simulink model "HARMALYZE_model_simulink"  (R2019b)
settings: Solver=VariableStepAuto  StartTime=0.0  StopTime=2.3  RelTol=1e-3
libraries: powerlib_meascontrol x1
(part 2 of 2)

== system HARMALYZE_model_simulink/Subsystem2/Subsystem1/An Bn finder ==
  signal : Inport
  pulse : Inport  Port=2
  cos : Inport  Port=3
  sin : Inport  Port=4
  "freq " : Inport  Port=5
  Add2 : Sum  Inputs=+-
  Constant1 : Constant  Value=0.0095
  Data Store Read1 : DataStoreRead  DataStoreName=simultion_time
  Product : Product  Inputs=3
  Product{1,3..5} (4 alike) : Product
  Product2 : Product  Inputs=3
  Pulse Generator1 : DiscretePulseGenerator  PulseType=Time based  Period=1  PulseWidth=0.01
  Transfer Fcn1 : TransferFcn  Numerator=[2]  Denominator=[1 0]
  Transfer Fcn2 : TransferFcn  Numerator=[2]  Denominator=[1 0]
  Variable Time Delay1 : VariableTransportDelay  MaximumDelay=10
  An : Outport
  Bn : Outport  Port=2
  wires:
  Product4/1 -> Bn/1
  Product5/1 -> An/1
  Product3/1 -> Product4/2  "Bn"
  Add2/1 -> Variable Time Delay1/2
  Variable Time Delay1/1 -> Product4/1, Product5/2
  Data Store Read1/1 -> Add2/1
  Constant1/1 -> Add2/2
  Product1/1 -> Product5/1  "An"
  Pulse Generator1/1 -> Variable Time Delay1/1
  "freq "/1 -> Product3/1, Product1/2
  Transfer Fcn1/1 -> Product1/1
  Transfer Fcn2/1 -> Product3/2
  sin/1 -> Product2/3
  cos/1 -> Product/3
  Product2/1 -> Transfer Fcn2/1
  Product/1 -> Transfer Fcn1/1
  signal/1 -> Product/2, Product2/1
  pulse/1 -> Product2/2, Product/1

== system HARMALYZE_model_simulink/Subsystem2/Subsystem1/magnitude ==
  An : Inport
  Bn : Inport  Port=2
  Add3 : Sum
  Math Function : Math  Operator=square  SignedPower=off  SaturateOnIntegerOverflow=on
  Math Function1 : Math  Operator=square  SignedPower=off  SaturateOnIntegerOverflow=on
  Sqrt : Sqrt  SaturateOnIntegerOverflow=on
  Out1 : Outport
  wires:
  An/1 -> Math Function/1
  Bn/1 -> Math Function1/1
  Sqrt/1 -> Out1/1
  Math Function1/1 -> Add3/2
  Add3/1 -> Sqrt/1
  Math Function/1 -> Add3/1

== system HARMALYZE_model_simulink/Subsystem2/Subsystem1/phase ==
  An : Inport
  Bn : Inport  Port=2
  Multiply1 : Gain  Gain=180/pi
  Sin : Trigonometry  Operator=atan2
  Out1 : Outport
  wires:
  Multiply1/1 -> Out1/1
  Bn/1 -> Sin/1
  An/1 -> Sin/2
  Sin/1 -> Multiply1/1

== system HARMALYZE_model_simulink/Subsystem2/Subsystem1/sin cos wave generator ==
  freq : Inport
  clock : Inport  Port=2
  Cos1 : Trigonometry  Operator=cos
  Gain : Gain  Gain=2*pi
  Product1 : Product
  Sin1 : Trigonometry
  cos : Outport
  sin : Outport  Port=2
  wires:
  Gain/1 -> Cos1/1, Sin1/1
  Product1/1 -> Gain/1
  Sin1/1 -> sin/1
  clock/1 -> Product1/2
  freq/1 -> Product1/1
  Cos1/1 -> cos/1

== system HARMALYZE_model_simulink/Subsystem2/Subsystem10/An Bn finder ==
  signal : Inport
  pulse : Inport  Port=2
  cos : Inport  Port=3
  sin : Inport  Port=4
  "freq " : Inport  Port=5
  Add2 : Sum  Inputs=+-
  Constant1 : Constant  Value=0.005
  Data Store Read1 : DataStoreRead  DataStoreName=simultion_time
  Product : Product  Inputs=3
  Product{1,3..5} (4 alike) : Product
  Product2 : Product  Inputs=3
  Pulse Generator1 : DiscretePulseGenerator  PulseType=Time based  Period=1  PulseWidth=0.01
  Transfer Fcn1 : TransferFcn  Numerator=[2]  Denominator=[1 0]
  Transfer Fcn2 : TransferFcn  Numerator=[2]  Denominator=[1 0]
  Variable Time Delay1 : VariableTransportDelay  MaximumDelay=10
  An : Outport
  Bn : Outport  Port=2
  wires:
  Product4/1 -> Bn/1
  Product5/1 -> An/1
  Product3/1 -> Product4/2  "Bn"
  Add2/1 -> Variable Time Delay1/2
  Variable Time Delay1/1 -> Product4/1, Product5/2
  Data Store Read1/1 -> Add2/1
  Constant1/1 -> Add2/2
  Product1/1 -> Product5/1  "An"
  Pulse Generator1/1 -> Variable Time Delay1/1
  "freq "/1 -> Product3/1, Product1/2
  Transfer Fcn1/1 -> Product1/1
  Transfer Fcn2/1 -> Product3/2
  sin/1 -> Product2/3
  cos/1 -> Product/3
  Product2/1 -> Transfer Fcn2/1
  Product/1 -> Transfer Fcn1/1
  signal/1 -> Product/2, Product2/1
  pulse/1 -> Product2/2, Product/1

== system HARMALYZE_model_simulink/Subsystem2/Subsystem10/magnitude ==
  An : Inport
  Bn : Inport  Port=2
  Add3 : Sum
  Math Function : Math  Operator=square  SignedPower=off  SaturateOnIntegerOverflow=on
  Math Function1 : Math  Operator=square  SignedPower=off  SaturateOnIntegerOverflow=on
  Sqrt : Sqrt  SaturateOnIntegerOverflow=on
  Out1 : Outport
  wires:
  An/1 -> Math Function/1
  Bn/1 -> Math Function1/1
  Sqrt/1 -> Out1/1
  Math Function1/1 -> Add3/2
  Add3/1 -> Sqrt/1
  Math Function/1 -> Add3/1

== system HARMALYZE_model_simulink/Subsystem2/Subsystem10/phase ==
  An : Inport
  Bn : Inport  Port=2
  Multiply1 : Gain  Gain=180/pi
  Sin : Trigonometry  Operator=atan2
  Out1 : Outport
  wires:
  Multiply1/1 -> Out1/1
  Bn/1 -> Sin/1
  An/1 -> Sin/2
  Sin/1 -> Multiply1/1

== system HARMALYZE_model_simulink/Subsystem2/Subsystem10/sin cos wave generator ==
  freq : Inport
  clock : Inport  Port=2
  Cos1 : Trigonometry  Operator=cos
  Gain : Gain  Gain=2*pi
  Product1 : Product
  Sin1 : Trigonometry
  cos : Outport
  sin : Outport  Port=2
  wires:
  Gain/1 -> Cos1/1, Sin1/1
  Product1/1 -> Gain/1
  Sin1/1 -> sin/1
  clock/1 -> Product1/2
  freq/1 -> Product1/1
  Cos1/1 -> cos/1

== system HARMALYZE_model_simulink/Subsystem2/Subsystem11/An Bn finder ==
  signal : Inport
  pulse : Inport  Port=2
  cos : Inport  Port=3
  sin : Inport  Port=4
  "freq " : Inport  Port=5
  Add2 : Sum  Inputs=+-
  Constant1 : Constant  Value=0.0015
  Data Store Read1 : DataStoreRead  DataStoreName=simultion_time
  Product : Product  Inputs=3
  Product{1,3..5} (4 alike) : Product
  Product2 : Product  Inputs=3
  Pulse Generator1 : DiscretePulseGenerator  PulseType=Time based  Period=1  PulseWidth=0.01
  Transfer Fcn1 : TransferFcn  Numerator=[2]  Denominator=[1 0]
  Transfer Fcn2 : TransferFcn  Numerator=[2]  Denominator=[1 0]
  Variable Time Delay1 : VariableTransportDelay  MaximumDelay=10
  An : Outport
  Bn : Outport  Port=2
  wires:
  pulse/1 -> Product/1, Product2/2
  signal/1 -> Product2/1, Product/2
  Product/1 -> Transfer Fcn1/1
  Product2/1 -> Transfer Fcn2/1
  cos/1 -> Product/3
  sin/1 -> Product2/3
  Transfer Fcn2/1 -> Product3/2
  Transfer Fcn1/1 -> Product1/1
  "freq "/1 -> Product1/2, Product3/1
  Pulse Generator1/1 -> Variable Time Delay1/1
  Product1/1 -> Product5/1  "An"
  Constant1/1 -> Add2/2
  Data Store Read1/1 -> Add2/1
  Variable Time Delay1/1 -> Product5/2, Product4/1
  Add2/1 -> Variable Time Delay1/2
  Product3/1 -> Product4/2  "Bn"
  Product5/1 -> An/1
  Product4/1 -> Bn/1

== system HARMALYZE_model_simulink/Subsystem2/Subsystem11/magnitude ==
  An : Inport
  Bn : Inport  Port=2
  Add3 : Sum
  Math Function : Math  Operator=square  SignedPower=off  SaturateOnIntegerOverflow=on
  Math Function1 : Math  Operator=square  SignedPower=off  SaturateOnIntegerOverflow=on
  Sqrt : Sqrt  SaturateOnIntegerOverflow=on
  Out1 : Outport
  wires:
  Math Function/1 -> Add3/1
  Add3/1 -> Sqrt/1
  Math Function1/1 -> Add3/2
  Sqrt/1 -> Out1/1
  Bn/1 -> Math Function1/1
  An/1 -> Math Function/1

== system HARMALYZE_model_simulink/Subsystem2/Subsystem11/phase ==
  An : Inport
  Bn : Inport  Port=2
  Multiply1 : Gain  Gain=180/pi
  Sin : Trigonometry  Operator=atan2
  Out1 : Outport
  wires:
  Sin/1 -> Multiply1/1
  An/1 -> Sin/2
  Bn/1 -> Sin/1
  Multiply1/1 -> Out1/1

== system HARMALYZE_model_simulink/Subsystem2/Subsystem11/sin cos wave generator ==
  freq : Inport
  clock : Inport  Port=2
  Cos1 : Trigonometry  Operator=cos
  Gain : Gain  Gain=2*pi
  Product1 : Product
  Sin1 : Trigonometry
  cos : Outport
  sin : Outport  Port=2
  wires:
  Cos1/1 -> cos/1
  freq/1 -> Product1/1
  clock/1 -> Product1/2
  Sin1/1 -> sin/1
  Product1/1 -> Gain/1
  Gain/1 -> Sin1/1, Cos1/1

== system HARMALYZE_model_simulink/Subsystem2/Subsystem12/An Bn finder ==
  signal : Inport
  pulse : Inport  Port=2
  cos : Inport  Port=3
  sin : Inport  Port=4
  "freq " : Inport  Port=5
  Add2 : Sum  Inputs=+-
  Constant1 : Constant  Value=0.0045
  Data Store Read1 : DataStoreRead  DataStoreName=simultion_time
  Product : Product  Inputs=3
  Product{1,3..5} (4 alike) : Product
  Product2 : Product  Inputs=3
  Pulse Generator1 : DiscretePulseGenerator  PulseType=Time based  Period=1  PulseWidth=0.01
  Transfer Fcn1 : TransferFcn  Numerator=[2]  Denominator=[1 0]
  Transfer Fcn2 : TransferFcn  Numerator=[2]  Denominator=[1 0]
  Variable Time Delay1 : VariableTransportDelay  MaximumDelay=10
  An : Outport
  Bn : Outport  Port=2
  wires:
  Product4/1 -> Bn/1
  Product5/1 -> An/1
  Product3/1 -> Product4/2  "Bn"
  Add2/1 -> Variable Time Delay1/2
  Variable Time Delay1/1 -> Product4/1, Product5/2
  Data Store Read1/1 -> Add2/1
  Constant1/1 -> Add2/2
  Product1/1 -> Product5/1  "An"
  Pulse Generator1/1 -> Variable Time Delay1/1
  "freq "/1 -> Product3/1, Product1/2
  Transfer Fcn1/1 -> Product1/1
  Transfer Fcn2/1 -> Product3/2
  sin/1 -> Product2/3
  cos/1 -> Product/3
  Product2/1 -> Transfer Fcn2/1
  Product/1 -> Transfer Fcn1/1
  signal/1 -> Product/2, Product2/1
  pulse/1 -> Product2/2, Product/1

== system HARMALYZE_model_simulink/Subsystem2/Subsystem12/magnitude ==
  An : Inport
  Bn : Inport  Port=2
  Add3 : Sum
  Math Function : Math  Operator=square  SignedPower=off  SaturateOnIntegerOverflow=on
  Math Function1 : Math  Operator=square  SignedPower=off  SaturateOnIntegerOverflow=on
  Sqrt : Sqrt  SaturateOnIntegerOverflow=on
  Out1 : Outport
  wires:
  An/1 -> Math Function/1
  Bn/1 -> Math Function1/1
  Sqrt/1 -> Out1/1
  Math Function1/1 -> Add3/2
  Add3/1 -> Sqrt/1
  Math Function/1 -> Add3/1

== system HARMALYZE_model_simulink/Subsystem2/Subsystem12/phase ==
  An : Inport
  Bn : Inport  Port=2
  Multiply1 : Gain  Gain=180/pi
  Sin : Trigonometry  Operator=atan2
  Out1 : Outport
  wires:
  Multiply1/1 -> Out1/1
  Bn/1 -> Sin/1
  An/1 -> Sin/2
  Sin/1 -> Multiply1/1

== system HARMALYZE_model_simulink/Subsystem2/Subsystem12/sin cos wave generator ==
  freq : Inport
  clock : Inport  Port=2
  Cos1 : Trigonometry  Operator=cos
  Gain : Gain  Gain=2*pi
  Product1 : Product
  Sin1 : Trigonometry
  cos : Outport
  sin : Outport  Port=2
  wires:
  Gain/1 -> Cos1/1, Sin1/1
  Product1/1 -> Gain/1
  Sin1/1 -> sin/1
  clock/1 -> Product1/2
  freq/1 -> Product1/1
  Cos1/1 -> cos/1

== system HARMALYZE_model_simulink/Subsystem2/Subsystem13/An Bn finder ==
  signal : Inport
  pulse : Inport  Port=2
  cos : Inport  Port=3
  sin : Inport  Port=4
  "freq " : Inport  Port=5
  Add2 : Sum  Inputs=+-
  Constant1 : Constant  Value=0.004
  Data Store Read1 : DataStoreRead  DataStoreName=simultion_time
  Product : Product  Inputs=3
  Product{1,3..5} (4 alike) : Product
  Product2 : Product  Inputs=3
  Pulse Generator1 : DiscretePulseGenerator  PulseType=Time based  Period=1  PulseWidth=0.01
  Transfer Fcn1 : TransferFcn  Numerator=[2]  Denominator=[1 0]
  Transfer Fcn2 : TransferFcn  Numerator=[2]  Denominator=[1 0]
  Variable Time Delay1 : VariableTransportDelay  MaximumDelay=10
  An : Outport
  Bn : Outport  Port=2
  wires:
  Product4/1 -> Bn/1
  Product5/1 -> An/1
  Product3/1 -> Product4/2  "Bn"
  Add2/1 -> Variable Time Delay1/2
  Variable Time Delay1/1 -> Product4/1, Product5/2
  Data Store Read1/1 -> Add2/1
  Constant1/1 -> Add2/2
  Product1/1 -> Product5/1  "An"
  Pulse Generator1/1 -> Variable Time Delay1/1
  "freq "/1 -> Product3/1, Product1/2
  Transfer Fcn1/1 -> Product1/1
  Transfer Fcn2/1 -> Product3/2
  sin/1 -> Product2/3
  cos/1 -> Product/3
  Product2/1 -> Transfer Fcn2/1
  Product/1 -> Transfer Fcn1/1
  signal/1 -> Product/2, Product2/1
  pulse/1 -> Product2/2, Product/1

== system HARMALYZE_model_simulink/Subsystem2/Subsystem13/magnitude ==
  An : Inport
  Bn : Inport  Port=2
  Add3 : Sum
  Math Function : Math  Operator=square  SignedPower=off  SaturateOnIntegerOverflow=on
  Math Function1 : Math  Operator=square  SignedPower=off  SaturateOnIntegerOverflow=on
  Sqrt : Sqrt  SaturateOnIntegerOverflow=on
  Out1 : Outport
  wires:
  An/1 -> Math Function/1
  Bn/1 -> Math Function1/1
  Sqrt/1 -> Out1/1
  Math Function1/1 -> Add3/2
  Add3/1 -> Sqrt/1
  Math Function/1 -> Add3/1

== system HARMALYZE_model_simulink/Subsystem2/Subsystem13/phase ==
  An : Inport
  Bn : Inport  Port=2
  Multiply1 : Gain  Gain=180/pi
  Sin : Trigonometry  Operator=atan2
  Out1 : Outport
  wires:
  Multiply1/1 -> Out1/1
  Bn/1 -> Sin/1
  An/1 -> Sin/2
  Sin/1 -> Multiply1/1

== system HARMALYZE_model_simulink/Subsystem2/Subsystem13/sin cos wave generator ==
  freq : Inport
  clock : Inport  Port=2
  Cos1 : Trigonometry  Operator=cos
  Gain : Gain  Gain=2*pi
  Product1 : Product
  Sin1 : Trigonometry
  cos : Outport
  sin : Outport  Port=2
  wires:
  Gain/1 -> Cos1/1, Sin1/1
  Product1/1 -> Gain/1
  Sin1/1 -> sin/1
  clock/1 -> Product1/2
  freq/1 -> Product1/1
  Cos1/1 -> cos/1

== system HARMALYZE_model_simulink/Subsystem2/Subsystem14/An Bn finder ==
  signal : Inport
  pulse : Inport  Port=2
  cos : Inport  Port=3
  sin : Inport  Port=4
  "freq " : Inport  Port=5
  Add2 : Sum  Inputs=+-
  Constant1 : Constant  Value=0.0035
  Data Store Read1 : DataStoreRead  DataStoreName=simultion_time
  Product : Product  Inputs=3
  Product{1,3..5} (4 alike) : Product
  Product2 : Product  Inputs=3
  Pulse Generator1 : DiscretePulseGenerator  PulseType=Time based  Period=1  PulseWidth=0.01
  Transfer Fcn1 : TransferFcn  Numerator=[2]  Denominator=[1 0]
  Transfer Fcn2 : TransferFcn  Numerator=[2]  Denominator=[1 0]
  Variable Time Delay1 : VariableTransportDelay  MaximumDelay=10
  An : Outport
  Bn : Outport  Port=2
  wires:
  Product4/1 -> Bn/1
  Product5/1 -> An/1
  Product3/1 -> Product4/2  "Bn"
  Add2/1 -> Variable Time Delay1/2
  Variable Time Delay1/1 -> Product4/1, Product5/2
  Data Store Read1/1 -> Add2/1
  Constant1/1 -> Add2/2
  Product1/1 -> Product5/1  "An"
  Pulse Generator1/1 -> Variable Time Delay1/1
  "freq "/1 -> Product3/1, Product1/2
  Transfer Fcn1/1 -> Product1/1
  Transfer Fcn2/1 -> Product3/2
  sin/1 -> Product2/3
  cos/1 -> Product/3
  Product2/1 -> Transfer Fcn2/1
  Product/1 -> Transfer Fcn1/1
  signal/1 -> Product/2, Product2/1
  pulse/1 -> Product2/2, Product/1

== system HARMALYZE_model_simulink/Subsystem2/Subsystem14/magnitude ==
  An : Inport
  Bn : Inport  Port=2
  Add3 : Sum
  Math Function : Math  Operator=square  SignedPower=off  SaturateOnIntegerOverflow=on
  Math Function1 : Math  Operator=square  SignedPower=off  SaturateOnIntegerOverflow=on
  Sqrt : Sqrt  SaturateOnIntegerOverflow=on
  Out1 : Outport
  wires:
  An/1 -> Math Function/1
  Bn/1 -> Math Function1/1
  Sqrt/1 -> Out1/1
  Math Function1/1 -> Add3/2
  Add3/1 -> Sqrt/1
  Math Function/1 -> Add3/1

== system HARMALYZE_model_simulink/Subsystem2/Subsystem14/phase ==
  An : Inport
  Bn : Inport  Port=2
  Multiply1 : Gain  Gain=180/pi
  Sin : Trigonometry  Operator=atan2
  Out1 : Outport
  wires:
  Multiply1/1 -> Out1/1
  Bn/1 -> Sin/1
  An/1 -> Sin/2
  Sin/1 -> Multiply1/1

== system HARMALYZE_model_simulink/Subsystem2/Subsystem14/sin cos wave generator ==
  freq : Inport
  clock : Inport  Port=2
  Cos1 : Trigonometry  Operator=cos
  Gain : Gain  Gain=2*pi
  Product1 : Product
  Sin1 : Trigonometry
  cos : Outport
  sin : Outport  Port=2
  wires:
  Gain/1 -> Cos1/1, Sin1/1
  Product1/1 -> Gain/1
  Sin1/1 -> sin/1
  clock/1 -> Product1/2
  freq/1 -> Product1/1
  Cos1/1 -> cos/1

== system HARMALYZE_model_simulink/Subsystem2/Subsystem15/An Bn finder ==
  signal : Inport
  pulse : Inport  Port=2
  cos : Inport  Port=3
  sin : Inport  Port=4
  "freq " : Inport  Port=5
  Add2 : Sum  Inputs=+-
  Constant1 : Constant  Value=0.003
  Data Store Read1 : DataStoreRead  DataStoreName=simultion_time
  Product : Product  Inputs=3
  Product{1,3..5} (4 alike) : Product
  Product2 : Product  Inputs=3
  Pulse Generator1 : DiscretePulseGenerator  PulseType=Time based  Period=1  PulseWidth=0.01
  Transfer Fcn1 : TransferFcn  Numerator=[2]  Denominator=[1 0]
  Transfer Fcn2 : TransferFcn  Numerator=[2]  Denominator=[1 0]
  Variable Time Delay1 : VariableTransportDelay  MaximumDelay=10
  An : Outport
  Bn : Outport  Port=2
  wires:
  Product4/1 -> Bn/1
  Product5/1 -> An/1
  Product3/1 -> Product4/2  "Bn"
  Add2/1 -> Variable Time Delay1/2
  Variable Time Delay1/1 -> Product4/1, Product5/2
  Data Store Read1/1 -> Add2/1
  Constant1/1 -> Add2/2
  Product1/1 -> Product5/1  "An"
  Pulse Generator1/1 -> Variable Time Delay1/1
  "freq "/1 -> Product3/1, Product1/2
  Transfer Fcn1/1 -> Product1/1
  Transfer Fcn2/1 -> Product3/2
  sin/1 -> Product2/3
  cos/1 -> Product/3
  Product2/1 -> Transfer Fcn2/1
  Product/1 -> Transfer Fcn1/1
  signal/1 -> Product/2, Product2/1
  pulse/1 -> Product2/2, Product/1

== system HARMALYZE_model_simulink/Subsystem2/Subsystem15/magnitude ==
  An : Inport
  Bn : Inport  Port=2
  Add3 : Sum
  Math Function : Math  Operator=square  SignedPower=off  SaturateOnIntegerOverflow=on
  Math Function1 : Math  Operator=square  SignedPower=off  SaturateOnIntegerOverflow=on
  Sqrt : Sqrt  SaturateOnIntegerOverflow=on
  Out1 : Outport
  wires:
  An/1 -> Math Function/1
  Bn/1 -> Math Function1/1
  Sqrt/1 -> Out1/1
  Math Function1/1 -> Add3/2
  Add3/1 -> Sqrt/1
  Math Function/1 -> Add3/1

== system HARMALYZE_model_simulink/Subsystem2/Subsystem15/phase ==
  An : Inport
  Bn : Inport  Port=2
  Multiply1 : Gain  Gain=180/pi
  Sin : Trigonometry  Operator=atan2
  Out1 : Outport
  wires:
  Multiply1/1 -> Out1/1
  Bn/1 -> Sin/1
  An/1 -> Sin/2
  Sin/1 -> Multiply1/1

== system HARMALYZE_model_simulink/Subsystem2/Subsystem15/sin cos wave generator ==
  freq : Inport
  clock : Inport  Port=2
  Cos1 : Trigonometry  Operator=cos
  Gain : Gain  Gain=2*pi
  Product1 : Product
  Sin1 : Trigonometry
  cos : Outport
  sin : Outport  Port=2
  wires:
  Gain/1 -> Cos1/1, Sin1/1
  Product1/1 -> Gain/1
  Sin1/1 -> sin/1
  clock/1 -> Product1/2
  freq/1 -> Product1/1
  Cos1/1 -> cos/1

== system HARMALYZE_model_simulink/Subsystem2/Subsystem16/An Bn finder ==
  signal : Inport
  pulse : Inport  Port=2
  cos : Inport  Port=3
  sin : Inport  Port=4
  "freq " : Inport  Port=5
  Add2 : Sum  Inputs=+-
  Constant1 : Constant  Value=0.0025
  Data Store Read1 : DataStoreRead  DataStoreName=simultion_time
  Product : Product  Inputs=3
  Product{1,3..5} (4 alike) : Product
  Product2 : Product  Inputs=3
  Pulse Generator1 : DiscretePulseGenerator  PulseType=Time based  Period=1  PulseWidth=0.01
  Transfer Fcn1 : TransferFcn  Numerator=[2]  Denominator=[1 0]
  Transfer Fcn2 : TransferFcn  Numerator=[2]  Denominator=[1 0]
  Variable Time Delay1 : VariableTransportDelay  MaximumDelay=10
  An : Outport
  Bn : Outport  Port=2
  wires:
  pulse/1 -> Product/1, Product2/2
  signal/1 -> Product2/1, Product/2
  Product/1 -> Transfer Fcn1/1
  Product2/1 -> Transfer Fcn2/1
  cos/1 -> Product/3
  sin/1 -> Product2/3
  Transfer Fcn2/1 -> Product3/2
  Transfer Fcn1/1 -> Product1/1
  "freq "/1 -> Product1/2, Product3/1
  Pulse Generator1/1 -> Variable Time Delay1/1
  Product1/1 -> Product5/1  "An"
  Constant1/1 -> Add2/2
  Data Store Read1/1 -> Add2/1
  Variable Time Delay1/1 -> Product5/2, Product4/1
  Add2/1 -> Variable Time Delay1/2
  Product3/1 -> Product4/2  "Bn"
  Product5/1 -> An/1
  Product4/1 -> Bn/1

== system HARMALYZE_model_simulink/Subsystem2/Subsystem16/magnitude ==
  An : Inport
  Bn : Inport  Port=2
  Add3 : Sum
  Math Function : Math  Operator=square  SignedPower=off  SaturateOnIntegerOverflow=on
  Math Function1 : Math  Operator=square  SignedPower=off  SaturateOnIntegerOverflow=on
  Sqrt : Sqrt  SaturateOnIntegerOverflow=on
  Out1 : Outport
  wires:
  Math Function/1 -> Add3/1
  Add3/1 -> Sqrt/1
  Math Function1/1 -> Add3/2
  Sqrt/1 -> Out1/1
  Bn/1 -> Math Function1/1
  An/1 -> Math Function/1

== system HARMALYZE_model_simulink/Subsystem2/Subsystem16/phase ==
  An : Inport
  Bn : Inport  Port=2
  Multiply1 : Gain  Gain=180/pi
  Sin : Trigonometry  Operator=atan2
  Out1 : Outport
  wires:
  Sin/1 -> Multiply1/1
  An/1 -> Sin/2
  Bn/1 -> Sin/1
  Multiply1/1 -> Out1/1

== system HARMALYZE_model_simulink/Subsystem2/Subsystem16/sin cos wave generator ==
  freq : Inport
  clock : Inport  Port=2
  Cos1 : Trigonometry  Operator=cos
  Gain : Gain  Gain=2*pi
  Product1 : Product
  Sin1 : Trigonometry
  cos : Outport
  sin : Outport  Port=2
  wires:
  Cos1/1 -> cos/1
  freq/1 -> Product1/1
  clock/1 -> Product1/2
  Sin1/1 -> sin/1
  Product1/1 -> Gain/1
  Gain/1 -> Sin1/1, Cos1/1

== system HARMALYZE_model_simulink/Subsystem2/Subsystem17/An Bn finder ==
  signal : Inport
  pulse : Inport  Port=2
  cos : Inport  Port=3
  sin : Inport  Port=4
  "freq " : Inport  Port=5
  Add2 : Sum  Inputs=+-
  Constant1 : Constant  Value=0.002
  Data Store Read1 : DataStoreRead  DataStoreName=simultion_time
  Product : Product  Inputs=3
  Product{1,3..5} (4 alike) : Product
  Product2 : Product  Inputs=3
  Pulse Generator1 : DiscretePulseGenerator  PulseType=Time based  Period=1  PulseWidth=0.01
  Transfer Fcn1 : TransferFcn  Numerator=[2]  Denominator=[1 0]
  Transfer Fcn2 : TransferFcn  Numerator=[2]  Denominator=[1 0]
  Variable Time Delay1 : VariableTransportDelay  MaximumDelay=10
  An : Outport
  Bn : Outport  Port=2
  wires:
  pulse/1 -> Product/1, Product2/2
  signal/1 -> Product2/1, Product/2
  Product/1 -> Transfer Fcn1/1
  Product2/1 -> Transfer Fcn2/1
  cos/1 -> Product/3
  sin/1 -> Product2/3
  Transfer Fcn2/1 -> Product3/2
  Transfer Fcn1/1 -> Product1/1
  "freq "/1 -> Product1/2, Product3/1
  Pulse Generator1/1 -> Variable Time Delay1/1
  Product1/1 -> Product5/1  "An"
  Constant1/1 -> Add2/2
  Data Store Read1/1 -> Add2/1
  Variable Time Delay1/1 -> Product5/2, Product4/1
  Add2/1 -> Variable Time Delay1/2
  Product3/1 -> Product4/2  "Bn"
  Product5/1 -> An/1
  Product4/1 -> Bn/1

== system HARMALYZE_model_simulink/Subsystem2/Subsystem17/magnitude ==
  An : Inport
  Bn : Inport  Port=2
  Add3 : Sum
  Math Function : Math  Operator=square  SignedPower=off  SaturateOnIntegerOverflow=on
  Math Function1 : Math  Operator=square  SignedPower=off  SaturateOnIntegerOverflow=on
  Sqrt : Sqrt  SaturateOnIntegerOverflow=on
  Out1 : Outport
  wires:
  Math Function/1 -> Add3/1
  Add3/1 -> Sqrt/1
  Math Function1/1 -> Add3/2
  Sqrt/1 -> Out1/1
  Bn/1 -> Math Function1/1
  An/1 -> Math Function/1

== system HARMALYZE_model_simulink/Subsystem2/Subsystem17/phase ==
  An : Inport
  Bn : Inport  Port=2
  Multiply1 : Gain  Gain=180/pi
  Sin : Trigonometry  Operator=atan2
  Out1 : Outport
  wires:
  Sin/1 -> Multiply1/1
  An/1 -> Sin/2
  Bn/1 -> Sin/1
  Multiply1/1 -> Out1/1

== system HARMALYZE_model_simulink/Subsystem2/Subsystem17/sin cos wave generator ==
  freq : Inport
  clock : Inport  Port=2
  Cos1 : Trigonometry  Operator=cos
  Gain : Gain  Gain=2*pi
  Product1 : Product
  Sin1 : Trigonometry
  cos : Outport
  sin : Outport  Port=2
  wires:
  Cos1/1 -> cos/1
  freq/1 -> Product1/1
  clock/1 -> Product1/2
  Sin1/1 -> sin/1
  Product1/1 -> Gain/1
  Gain/1 -> Sin1/1, Cos1/1

== system HARMALYZE_model_simulink/Subsystem2/Subsystem18/An Bn finder ==
  signal : Inport
  pulse : Inport  Port=2
  cos : Inport  Port=3
  sin : Inport  Port=4
  "freq " : Inport  Port=5
  Add2 : Sum  Inputs=+-
  Constant1 : Constant  Value=0.0005
  Data Store Read1 : DataStoreRead  DataStoreName=simultion_time
  Product : Product  Inputs=3
  Product{1,3..5} (4 alike) : Product
  Product2 : Product  Inputs=3
  Pulse Generator1 : DiscretePulseGenerator  PulseType=Time based  Period=1  PulseWidth=0.01
  Transfer Fcn1 : TransferFcn  Numerator=[2]  Denominator=[1 0]
  Transfer Fcn2 : TransferFcn  Numerator=[2]  Denominator=[1 0]
  Variable Time Delay1 : VariableTransportDelay  MaximumDelay=10
  An : Outport
  Bn : Outport  Port=2
  wires:
  Product4/1 -> Bn/1
  Product5/1 -> An/1
  Product3/1 -> Product4/2  "Bn"
  Add2/1 -> Variable Time Delay1/2
  Variable Time Delay1/1 -> Product4/1, Product5/2
  Data Store Read1/1 -> Add2/1
  Constant1/1 -> Add2/2
  Product1/1 -> Product5/1  "An"
  Pulse Generator1/1 -> Variable Time Delay1/1
  "freq "/1 -> Product3/1, Product1/2
  Transfer Fcn1/1 -> Product1/1
  Transfer Fcn2/1 -> Product3/2
  sin/1 -> Product2/3
  cos/1 -> Product/3
  Product2/1 -> Transfer Fcn2/1
  Product/1 -> Transfer Fcn1/1
  signal/1 -> Product/2, Product2/1
  pulse/1 -> Product2/2, Product/1

== system HARMALYZE_model_simulink/Subsystem2/Subsystem18/magnitude ==
  An : Inport
  Bn : Inport  Port=2
  Add3 : Sum
  Math Function : Math  Operator=square  SignedPower=off  SaturateOnIntegerOverflow=on
  Math Function1 : Math  Operator=square  SignedPower=off  SaturateOnIntegerOverflow=on
  Sqrt : Sqrt  SaturateOnIntegerOverflow=on
  Out1 : Outport
  wires:
  An/1 -> Math Function/1
  Bn/1 -> Math Function1/1
  Sqrt/1 -> Out1/1
  Math Function1/1 -> Add3/2
  Add3/1 -> Sqrt/1
  Math Function/1 -> Add3/1

== system HARMALYZE_model_simulink/Subsystem2/Subsystem18/phase ==
  An : Inport
  Bn : Inport  Port=2
  Multiply1 : Gain  Gain=180/pi
  Sin : Trigonometry  Operator=atan2
  Out1 : Outport
  wires:
  Multiply1/1 -> Out1/1
  Bn/1 -> Sin/1
  An/1 -> Sin/2
  Sin/1 -> Multiply1/1

== system HARMALYZE_model_simulink/Subsystem2/Subsystem18/sin cos wave generator ==
  freq : Inport
  clock : Inport  Port=2
  Cos1 : Trigonometry  Operator=cos
  Gain : Gain  Gain=2*pi
  Product1 : Product
  Sin1 : Trigonometry
  cos : Outport
  sin : Outport  Port=2
  wires:
  Gain/1 -> Cos1/1, Sin1/1
  Product1/1 -> Gain/1
  Sin1/1 -> sin/1
  clock/1 -> Product1/2
  freq/1 -> Product1/1
  Cos1/1 -> cos/1

== system HARMALYZE_model_simulink/Subsystem2/Subsystem19/An Bn finder ==
  signal : Inport
  pulse : Inport  Port=2
  cos : Inport  Port=3
  sin : Inport  Port=4
  "freq " : Inport  Port=5
  Add2 : Sum  Inputs=+-
  Constant1 : Constant  Value=0.001
  Data Store Read1 : DataStoreRead  DataStoreName=simultion_time
  Product : Product  Inputs=3
  Product{1,3..5} (4 alike) : Product
  Product2 : Product  Inputs=3
  Pulse Generator1 : DiscretePulseGenerator  PulseType=Time based  Period=1  PulseWidth=0.01
  Transfer Fcn1 : TransferFcn  Numerator=[2]  Denominator=[1 0]
  Transfer Fcn2 : TransferFcn  Numerator=[2]  Denominator=[1 0]
  Variable Time Delay1 : VariableTransportDelay  MaximumDelay=10
  An : Outport
  Bn : Outport  Port=2
  wires:
  Product4/1 -> Bn/1
  Product5/1 -> An/1
  Product3/1 -> Product4/2  "Bn"
  Add2/1 -> Variable Time Delay1/2
  Variable Time Delay1/1 -> Product4/1, Product5/2
  Data Store Read1/1 -> Add2/1
  Constant1/1 -> Add2/2
  Product1/1 -> Product5/1  "An"
  Pulse Generator1/1 -> Variable Time Delay1/1
  "freq "/1 -> Product3/1, Product1/2
  Transfer Fcn1/1 -> Product1/1
  Transfer Fcn2/1 -> Product3/2
  sin/1 -> Product2/3
  cos/1 -> Product/3
  Product2/1 -> Transfer Fcn2/1
  Product/1 -> Transfer Fcn1/1
  signal/1 -> Product/2, Product2/1
  pulse/1 -> Product2/2, Product/1

== system HARMALYZE_model_simulink/Subsystem2/Subsystem19/magnitude ==
  An : Inport
  Bn : Inport  Port=2
  Add3 : Sum
  Math Function : Math  Operator=square  SignedPower=off  SaturateOnIntegerOverflow=on
  Math Function1 : Math  Operator=square  SignedPower=off  SaturateOnIntegerOverflow=on
  Sqrt : Sqrt  SaturateOnIntegerOverflow=on
  Out1 : Outport
  wires:
  An/1 -> Math Function/1
  Bn/1 -> Math Function1/1
  Sqrt/1 -> Out1/1
  Math Function1/1 -> Add3/2
  Add3/1 -> Sqrt/1
  Math Function/1 -> Add3/1

== system HARMALYZE_model_simulink/Subsystem2/Subsystem19/phase ==
  An : Inport
  Bn : Inport  Port=2
  Multiply1 : Gain  Gain=180/pi
  Sin : Trigonometry  Operator=atan2
  Out1 : Outport
  wires:
  Multiply1/1 -> Out1/1
  Bn/1 -> Sin/1
  An/1 -> Sin/2
  Sin/1 -> Multiply1/1

== system HARMALYZE_model_simulink/Subsystem2/Subsystem19/sin cos wave generator ==
  freq : Inport
  clock : Inport  Port=2
  Cos1 : Trigonometry  Operator=cos
  Gain : Gain  Gain=2*pi
  Product1 : Product
  Sin1 : Trigonometry
  cos : Outport
  sin : Outport  Port=2
  wires:
  Gain/1 -> Cos1/1, Sin1/1
  Product1/1 -> Gain/1
  Sin1/1 -> sin/1
  clock/1 -> Product1/2
  freq/1 -> Product1/1
  Cos1/1 -> cos/1

== system HARMALYZE_model_simulink/Subsystem2/Subsystem2/An Bn finder ==
  signal : Inport
  pulse : Inport  Port=2
  cos : Inport  Port=3
  sin : Inport  Port=4
  "freq " : Inport  Port=5
  Add2 : Sum  Inputs=+-
  Constant1 : Constant  Value=0.009
  Data Store Read1 : DataStoreRead  DataStoreName=simultion_time
  Product : Product  Inputs=3
  Product{1,3..5} (4 alike) : Product
  Product2 : Product  Inputs=3
  Pulse Generator1 : DiscretePulseGenerator  PulseType=Time based  Period=1  PulseWidth=0.01
  Transfer Fcn1 : TransferFcn  Numerator=[2]  Denominator=[1 0]
  Transfer Fcn2 : TransferFcn  Numerator=[2]  Denominator=[1 0]
  Variable Time Delay1 : VariableTransportDelay  MaximumDelay=10
  An : Outport
  Bn : Outport  Port=2
  wires:
  pulse/1 -> Product/1, Product2/2
  signal/1 -> Product2/1, Product/2
  Product/1 -> Transfer Fcn1/1
  Product2/1 -> Transfer Fcn2/1
  cos/1 -> Product/3
  sin/1 -> Product2/3
  Transfer Fcn2/1 -> Product3/2
  Transfer Fcn1/1 -> Product1/1
  "freq "/1 -> Product1/2, Product3/1
  Pulse Generator1/1 -> Variable Time Delay1/1
  Product1/1 -> Product5/1  "An"
  Constant1/1 -> Add2/2
  Data Store Read1/1 -> Add2/1
  Variable Time Delay1/1 -> Product5/2, Product4/1
  Add2/1 -> Variable Time Delay1/2
  Product3/1 -> Product4/2  "Bn"
  Product5/1 -> An/1
  Product4/1 -> Bn/1

== system HARMALYZE_model_simulink/Subsystem2/Subsystem2/magnitude ==
  An : Inport
  Bn : Inport  Port=2
  Add3 : Sum
  Math Function : Math  Operator=square  SignedPower=off  SaturateOnIntegerOverflow=on
  Math Function1 : Math  Operator=square  SignedPower=off  SaturateOnIntegerOverflow=on
  Sqrt : Sqrt  SaturateOnIntegerOverflow=on
  Out1 : Outport
  wires:
  Math Function/1 -> Add3/1
  Add3/1 -> Sqrt/1
  Math Function1/1 -> Add3/2
  Sqrt/1 -> Out1/1
  Bn/1 -> Math Function1/1
  An/1 -> Math Function/1

== system HARMALYZE_model_simulink/Subsystem2/Subsystem2/phase ==
  An : Inport
  Bn : Inport  Port=2
  Multiply1 : Gain  Gain=180/pi
  Sin : Trigonometry  Operator=atan2
  Out1 : Outport
  wires:
  Sin/1 -> Multiply1/1
  An/1 -> Sin/2
  Bn/1 -> Sin/1
  Multiply1/1 -> Out1/1

== system HARMALYZE_model_simulink/Subsystem2/Subsystem2/sin cos wave generator ==
  freq : Inport
  clock : Inport  Port=2
  Cos1 : Trigonometry  Operator=cos
  Gain : Gain  Gain=2*pi
  Product1 : Product
  Sin1 : Trigonometry
  cos : Outport
  sin : Outport  Port=2
  wires:
  Cos1/1 -> cos/1
  freq/1 -> Product1/1
  clock/1 -> Product1/2
  Sin1/1 -> sin/1
  Product1/1 -> Gain/1
  Gain/1 -> Sin1/1, Cos1/1

== system HARMALYZE_model_simulink/Subsystem2/Subsystem3/An Bn finder ==
  signal : Inport
  pulse : Inport  Port=2
  cos : Inport  Port=3
  sin : Inport  Port=4
  "freq " : Inport  Port=5
  Add2 : Sum  Inputs=+-
  Constant1 : Constant  Value=0.0085
  Data Store Read1 : DataStoreRead  DataStoreName=simultion_time
  Product : Product  Inputs=3
  Product{1,3..5} (4 alike) : Product
  Product2 : Product  Inputs=3
  Pulse Generator1 : DiscretePulseGenerator  PulseType=Time based  Period=1  PulseWidth=0.01
  Transfer Fcn1 : TransferFcn  Numerator=[2]  Denominator=[1 0]
  Transfer Fcn2 : TransferFcn  Numerator=[2]  Denominator=[1 0]
  Variable Time Delay1 : VariableTransportDelay  MaximumDelay=10
  An : Outport
  Bn : Outport  Port=2
  wires:
  Product4/1 -> Bn/1
  Product5/1 -> An/1
  Product3/1 -> Product4/2  "Bn"
  Add2/1 -> Variable Time Delay1/2
  Variable Time Delay1/1 -> Product4/1, Product5/2
  Data Store Read1/1 -> Add2/1
  Constant1/1 -> Add2/2
  Product1/1 -> Product5/1  "An"
  Pulse Generator1/1 -> Variable Time Delay1/1
  "freq "/1 -> Product3/1, Product1/2
  Transfer Fcn1/1 -> Product1/1
  Transfer Fcn2/1 -> Product3/2
  sin/1 -> Product2/3
  cos/1 -> Product/3
  Product2/1 -> Transfer Fcn2/1
  Product/1 -> Transfer Fcn1/1
  signal/1 -> Product/2, Product2/1
  pulse/1 -> Product2/2, Product/1

== system HARMALYZE_model_simulink/Subsystem2/Subsystem3/magnitude ==
  An : Inport
  Bn : Inport  Port=2
  Add3 : Sum
  Math Function : Math  Operator=square  SignedPower=off  SaturateOnIntegerOverflow=on
  Math Function1 : Math  Operator=square  SignedPower=off  SaturateOnIntegerOverflow=on
  Sqrt : Sqrt  SaturateOnIntegerOverflow=on
  Out1 : Outport
  wires:
  An/1 -> Math Function/1
  Bn/1 -> Math Function1/1
  Sqrt/1 -> Out1/1
  Math Function1/1 -> Add3/2
  Add3/1 -> Sqrt/1
  Math Function/1 -> Add3/1

== system HARMALYZE_model_simulink/Subsystem2/Subsystem3/phase ==
  An : Inport
  Bn : Inport  Port=2
  Multiply1 : Gain  Gain=180/pi
  Sin : Trigonometry  Operator=atan2
  Out1 : Outport
  wires:
  Multiply1/1 -> Out1/1
  Bn/1 -> Sin/1
  An/1 -> Sin/2
  Sin/1 -> Multiply1/1

== system HARMALYZE_model_simulink/Subsystem2/Subsystem3/sin cos wave generator ==
  freq : Inport
  clock : Inport  Port=2
  Cos1 : Trigonometry  Operator=cos
  Gain : Gain  Gain=2*pi
  Product1 : Product
  Sin1 : Trigonometry
  cos : Outport
  sin : Outport  Port=2
  wires:
  Gain/1 -> Cos1/1, Sin1/1
  Product1/1 -> Gain/1
  Sin1/1 -> sin/1
  clock/1 -> Product1/2
  freq/1 -> Product1/1
  Cos1/1 -> cos/1

== system HARMALYZE_model_simulink/Subsystem2/Subsystem4/An Bn finder ==
  signal : Inport
  pulse : Inport  Port=2
  cos : Inport  Port=3
  sin : Inport  Port=4
  "freq " : Inport  Port=5
  Add2 : Sum  Inputs=+-
  Constant1 : Constant  Value=0.008
  Data Store Read1 : DataStoreRead  DataStoreName=simultion_time
  Product : Product  Inputs=3
  Product{1,3..5} (4 alike) : Product
  Product2 : Product  Inputs=3
  Pulse Generator1 : DiscretePulseGenerator  PulseType=Time based  Period=1  PulseWidth=0.01
  Transfer Fcn1 : TransferFcn  Numerator=[2]  Denominator=[1 0]
  Transfer Fcn2 : TransferFcn  Numerator=[2]  Denominator=[1 0]
  Variable Time Delay1 : VariableTransportDelay  MaximumDelay=10
  An : Outport
  Bn : Outport  Port=2
  wires:
  pulse/1 -> Product/1, Product2/2
  signal/1 -> Product2/1, Product/2
  Product/1 -> Transfer Fcn1/1
  Product2/1 -> Transfer Fcn2/1
  cos/1 -> Product/3
  sin/1 -> Product2/3
  Transfer Fcn2/1 -> Product3/2
  Transfer Fcn1/1 -> Product1/1
  "freq "/1 -> Product1/2, Product3/1
  Pulse Generator1/1 -> Variable Time Delay1/1
  Product1/1 -> Product5/1  "An"
  Constant1/1 -> Add2/2
  Data Store Read1/1 -> Add2/1
  Variable Time Delay1/1 -> Product5/2, Product4/1
  Add2/1 -> Variable Time Delay1/2
  Product3/1 -> Product4/2  "Bn"
  Product5/1 -> An/1
  Product4/1 -> Bn/1

== system HARMALYZE_model_simulink/Subsystem2/Subsystem4/magnitude ==
  An : Inport
  Bn : Inport  Port=2
  Add3 : Sum
  Math Function : Math  Operator=square  SignedPower=off  SaturateOnIntegerOverflow=on
  Math Function1 : Math  Operator=square  SignedPower=off  SaturateOnIntegerOverflow=on
  Sqrt : Sqrt  SaturateOnIntegerOverflow=on
  Out1 : Outport
  wires:
  Math Function/1 -> Add3/1
  Add3/1 -> Sqrt/1
  Math Function1/1 -> Add3/2
  Sqrt/1 -> Out1/1
  Bn/1 -> Math Function1/1
  An/1 -> Math Function/1

== system HARMALYZE_model_simulink/Subsystem2/Subsystem4/phase ==
  An : Inport
  Bn : Inport  Port=2
  Multiply1 : Gain  Gain=180/pi
  Sin : Trigonometry  Operator=atan2
  Out1 : Outport
  wires:
  Sin/1 -> Multiply1/1
  An/1 -> Sin/2
  Bn/1 -> Sin/1
  Multiply1/1 -> Out1/1

== system HARMALYZE_model_simulink/Subsystem2/Subsystem4/sin cos wave generator ==
  freq : Inport
  clock : Inport  Port=2
  Cos1 : Trigonometry  Operator=cos
  Gain : Gain  Gain=2*pi
  Product1 : Product
  Sin1 : Trigonometry
  cos : Outport
  sin : Outport  Port=2
  wires:
  Cos1/1 -> cos/1
  freq/1 -> Product1/1
  clock/1 -> Product1/2
  Sin1/1 -> sin/1
  Product1/1 -> Gain/1
  Gain/1 -> Sin1/1, Cos1/1

== system HARMALYZE_model_simulink/Subsystem2/Subsystem5/An Bn finder ==
  signal : Inport
  pulse : Inport  Port=2
  cos : Inport  Port=3
  sin : Inport  Port=4
  "freq " : Inport  Port=5
  Add2 : Sum  Inputs=+-
  Constant1 : Constant  Value=0.0075
  Data Store Read1 : DataStoreRead  DataStoreName=simultion_time
  Product : Product  Inputs=3
  Product{1,3..5} (4 alike) : Product
  Product2 : Product  Inputs=3
  Pulse Generator1 : DiscretePulseGenerator  PulseType=Time based  Period=1  PulseWidth=0.01
  Transfer Fcn1 : TransferFcn  Numerator=[2]  Denominator=[1 0]
  Transfer Fcn2 : TransferFcn  Numerator=[2]  Denominator=[1 0]
  Variable Time Delay1 : VariableTransportDelay  MaximumDelay=10
  An : Outport
  Bn : Outport  Port=2
  wires:
  pulse/1 -> Product/1, Product2/2
  signal/1 -> Product2/1, Product/2
  Product/1 -> Transfer Fcn1/1
  Product2/1 -> Transfer Fcn2/1
  cos/1 -> Product/3
  sin/1 -> Product2/3
  Transfer Fcn2/1 -> Product3/2
  Transfer Fcn1/1 -> Product1/1
  "freq "/1 -> Product1/2, Product3/1
  Pulse Generator1/1 -> Variable Time Delay1/1
  Product1/1 -> Product5/1  "An"
  Constant1/1 -> Add2/2
  Data Store Read1/1 -> Add2/1
  Variable Time Delay1/1 -> Product5/2, Product4/1
  Add2/1 -> Variable Time Delay1/2
  Product3/1 -> Product4/2  "Bn"
  Product5/1 -> An/1
  Product4/1 -> Bn/1

== system HARMALYZE_model_simulink/Subsystem2/Subsystem5/magnitude ==
  An : Inport
  Bn : Inport  Port=2
  Add3 : Sum
  Math Function : Math  Operator=square  SignedPower=off  SaturateOnIntegerOverflow=on
  Math Function1 : Math  Operator=square  SignedPower=off  SaturateOnIntegerOverflow=on
  Sqrt : Sqrt  SaturateOnIntegerOverflow=on
  Out1 : Outport
  wires:
  Math Function/1 -> Add3/1
  Add3/1 -> Sqrt/1
  Math Function1/1 -> Add3/2
  Sqrt/1 -> Out1/1
  Bn/1 -> Math Function1/1
  An/1 -> Math Function/1

== system HARMALYZE_model_simulink/Subsystem2/Subsystem5/phase ==
  An : Inport
  Bn : Inport  Port=2
  Multiply1 : Gain  Gain=180/pi
  Sin : Trigonometry  Operator=atan2
  Out1 : Outport
  wires:
  Sin/1 -> Multiply1/1
  An/1 -> Sin/2
  Bn/1 -> Sin/1
  Multiply1/1 -> Out1/1

== system HARMALYZE_model_simulink/Subsystem2/Subsystem5/sin cos wave generator ==
  freq : Inport
  clock : Inport  Port=2
  Cos1 : Trigonometry  Operator=cos
  Gain : Gain  Gain=2*pi
  Product1 : Product
  Sin1 : Trigonometry
  cos : Outport
  sin : Outport  Port=2
  wires:
  Cos1/1 -> cos/1
  freq/1 -> Product1/1
  clock/1 -> Product1/2
  Sin1/1 -> sin/1
  Product1/1 -> Gain/1
  Gain/1 -> Sin1/1, Cos1/1

== system HARMALYZE_model_simulink/Subsystem2/Subsystem6/An Bn finder ==
  signal : Inport
  pulse : Inport  Port=2
  cos : Inport  Port=3
  sin : Inport  Port=4
  "freq " : Inport  Port=5
  Add2 : Sum  Inputs=+-
  Constant1 : Constant  Value=0.007
  Data Store Read1 : DataStoreRead  DataStoreName=simultion_time
  Product : Product  Inputs=3
  Product{1,3..5} (4 alike) : Product
  Product2 : Product  Inputs=3
  Pulse Generator1 : DiscretePulseGenerator  PulseType=Time based  Period=1  PulseWidth=0.01
  Transfer Fcn1 : TransferFcn  Numerator=[2]  Denominator=[1 0]
  Transfer Fcn2 : TransferFcn  Numerator=[2]  Denominator=[1 0]
  Variable Time Delay1 : VariableTransportDelay  MaximumDelay=10
  An : Outport
  Bn : Outport  Port=2
  wires:
  pulse/1 -> Product/1, Product2/2
  signal/1 -> Product2/1, Product/2
  Product/1 -> Transfer Fcn1/1
  Product2/1 -> Transfer Fcn2/1
  cos/1 -> Product/3
  sin/1 -> Product2/3
  Transfer Fcn2/1 -> Product3/2
  Transfer Fcn1/1 -> Product1/1
  "freq "/1 -> Product1/2, Product3/1
  Pulse Generator1/1 -> Variable Time Delay1/1
  Product1/1 -> Product5/1  "An"
  Constant1/1 -> Add2/2
  Data Store Read1/1 -> Add2/1
  Variable Time Delay1/1 -> Product5/2, Product4/1
  Add2/1 -> Variable Time Delay1/2
  Product3/1 -> Product4/2  "Bn"
  Product5/1 -> An/1
  Product4/1 -> Bn/1

== system HARMALYZE_model_simulink/Subsystem2/Subsystem6/magnitude ==
  An : Inport
  Bn : Inport  Port=2
  Add3 : Sum
  Math Function : Math  Operator=square  SignedPower=off  SaturateOnIntegerOverflow=on
  Math Function1 : Math  Operator=square  SignedPower=off  SaturateOnIntegerOverflow=on
  Sqrt : Sqrt  SaturateOnIntegerOverflow=on
  Out1 : Outport
  wires:
  Math Function/1 -> Add3/1
  Add3/1 -> Sqrt/1
  Math Function1/1 -> Add3/2
  Sqrt/1 -> Out1/1
  Bn/1 -> Math Function1/1
  An/1 -> Math Function/1

== system HARMALYZE_model_simulink/Subsystem2/Subsystem6/phase ==
  An : Inport
  Bn : Inport  Port=2
  Multiply1 : Gain  Gain=180/pi
  Sin : Trigonometry  Operator=atan2
  Out1 : Outport
  wires:
  Sin/1 -> Multiply1/1
  An/1 -> Sin/2
  Bn/1 -> Sin/1
  Multiply1/1 -> Out1/1

== system HARMALYZE_model_simulink/Subsystem2/Subsystem6/sin cos wave generator ==
  freq : Inport
  clock : Inport  Port=2
  Cos1 : Trigonometry  Operator=cos
  Gain : Gain  Gain=2*pi
  Product1 : Product
  Sin1 : Trigonometry
  cos : Outport
  sin : Outport  Port=2
  wires:
  Cos1/1 -> cos/1
  freq/1 -> Product1/1
  clock/1 -> Product1/2
  Sin1/1 -> sin/1
  Product1/1 -> Gain/1
  Gain/1 -> Sin1/1, Cos1/1

== system HARMALYZE_model_simulink/Subsystem2/Subsystem7/An Bn finder ==
  signal : Inport
  pulse : Inport  Port=2
  cos : Inport  Port=3
  sin : Inport  Port=4
  "freq " : Inport  Port=5
  Add2 : Sum  Inputs=+-
  Constant1 : Constant  Value=0.0065
  Data Store Read1 : DataStoreRead  DataStoreName=simultion_time
  Product : Product  Inputs=3
  Product{1,3..5} (4 alike) : Product
  Product2 : Product  Inputs=3
  Pulse Generator1 : DiscretePulseGenerator  PulseType=Time based  Period=1  PulseWidth=0.01
  Transfer Fcn1 : TransferFcn  Numerator=[2]  Denominator=[1 0]
  Transfer Fcn2 : TransferFcn  Numerator=[2]  Denominator=[1 0]
  Variable Time Delay1 : VariableTransportDelay  MaximumDelay=10
  An : Outport
  Bn : Outport  Port=2
  wires:
  pulse/1 -> Product/1, Product2/2
  signal/1 -> Product2/1, Product/2
  Product/1 -> Transfer Fcn1/1
  Product2/1 -> Transfer Fcn2/1
  cos/1 -> Product/3
  sin/1 -> Product2/3
  Transfer Fcn2/1 -> Product3/2
  Transfer Fcn1/1 -> Product1/1
  "freq "/1 -> Product1/2, Product3/1
  Pulse Generator1/1 -> Variable Time Delay1/1
  Product1/1 -> Product5/1  "An"
  Constant1/1 -> Add2/2
  Data Store Read1/1 -> Add2/1
  Variable Time Delay1/1 -> Product5/2, Product4/1
  Add2/1 -> Variable Time Delay1/2
  Product3/1 -> Product4/2  "Bn"
  Product5/1 -> An/1
  Product4/1 -> Bn/1

== system HARMALYZE_model_simulink/Subsystem2/Subsystem7/magnitude ==
  An : Inport
  Bn : Inport  Port=2
  Add3 : Sum
  Math Function : Math  Operator=square  SignedPower=off  SaturateOnIntegerOverflow=on
  Math Function1 : Math  Operator=square  SignedPower=off  SaturateOnIntegerOverflow=on
  Sqrt : Sqrt  SaturateOnIntegerOverflow=on
  Out1 : Outport
  wires:
  Math Function/1 -> Add3/1
  Add3/1 -> Sqrt/1
  Math Function1/1 -> Add3/2
  Sqrt/1 -> Out1/1
  Bn/1 -> Math Function1/1
  An/1 -> Math Function/1

== system HARMALYZE_model_simulink/Subsystem2/Subsystem7/phase ==
  An : Inport
  Bn : Inport  Port=2
  Multiply1 : Gain  Gain=180/pi
  Sin : Trigonometry  Operator=atan2
  Out1 : Outport
  wires:
  Sin/1 -> Multiply1/1
  An/1 -> Sin/2
  Bn/1 -> Sin/1
  Multiply1/1 -> Out1/1

== system HARMALYZE_model_simulink/Subsystem2/Subsystem7/sin cos wave generator ==
  freq : Inport
  clock : Inport  Port=2
  Cos1 : Trigonometry  Operator=cos
  Gain : Gain  Gain=2*pi
  Product1 : Product
  Sin1 : Trigonometry
  cos : Outport
  sin : Outport  Port=2
  wires:
  Cos1/1 -> cos/1
  freq/1 -> Product1/1
  clock/1 -> Product1/2
  Sin1/1 -> sin/1
  Product1/1 -> Gain/1
  Gain/1 -> Sin1/1, Cos1/1

== system HARMALYZE_model_simulink/Subsystem2/Subsystem8/An Bn finder ==
  signal : Inport
  pulse : Inport  Port=2
  cos : Inport  Port=3
  sin : Inport  Port=4
  "freq " : Inport  Port=5
  Add2 : Sum  Inputs=+-
  Constant1 : Constant  Value=0.006
  Data Store Read1 : DataStoreRead  DataStoreName=simultion_time
  Product : Product  Inputs=3
  Product{1,3..5} (4 alike) : Product
  Product2 : Product  Inputs=3
  Pulse Generator1 : DiscretePulseGenerator  PulseType=Time based  Period=1  PulseWidth=0.01
  Transfer Fcn1 : TransferFcn  Numerator=[2]  Denominator=[1 0]
  Transfer Fcn2 : TransferFcn  Numerator=[2]  Denominator=[1 0]
  Variable Time Delay1 : VariableTransportDelay  MaximumDelay=10
  An : Outport
  Bn : Outport  Port=2
  wires:
  Product4/1 -> Bn/1
  Product5/1 -> An/1
  Product3/1 -> Product4/2  "Bn"
  Add2/1 -> Variable Time Delay1/2
  Variable Time Delay1/1 -> Product4/1, Product5/2
  Data Store Read1/1 -> Add2/1
  Constant1/1 -> Add2/2
  Product1/1 -> Product5/1  "An"
  Pulse Generator1/1 -> Variable Time Delay1/1
  "freq "/1 -> Product3/1, Product1/2
  Transfer Fcn1/1 -> Product1/1
  Transfer Fcn2/1 -> Product3/2
  sin/1 -> Product2/3
  cos/1 -> Product/3
  Product2/1 -> Transfer Fcn2/1
  Product/1 -> Transfer Fcn1/1
  signal/1 -> Product/2, Product2/1
  pulse/1 -> Product2/2, Product/1

== system HARMALYZE_model_simulink/Subsystem2/Subsystem8/magnitude ==
  An : Inport
  Bn : Inport  Port=2
  Add3 : Sum
  Math Function : Math  Operator=square  SignedPower=off  SaturateOnIntegerOverflow=on
  Math Function1 : Math  Operator=square  SignedPower=off  SaturateOnIntegerOverflow=on
  Sqrt : Sqrt  SaturateOnIntegerOverflow=on
  Out1 : Outport
  wires:
  An/1 -> Math Function/1
  Bn/1 -> Math Function1/1
  Sqrt/1 -> Out1/1
  Math Function1/1 -> Add3/2
  Add3/1 -> Sqrt/1
  Math Function/1 -> Add3/1

== system HARMALYZE_model_simulink/Subsystem2/Subsystem8/phase ==
  An : Inport
  Bn : Inport  Port=2
  Multiply1 : Gain  Gain=180/pi
  Sin : Trigonometry  Operator=atan2
  Out1 : Outport
  wires:
  Multiply1/1 -> Out1/1
  Bn/1 -> Sin/1
  An/1 -> Sin/2
  Sin/1 -> Multiply1/1

== system HARMALYZE_model_simulink/Subsystem2/Subsystem8/sin cos wave generator ==
  freq : Inport
  clock : Inport  Port=2
  Cos1 : Trigonometry  Operator=cos
  Gain : Gain  Gain=2*pi
  Product1 : Product
  Sin1 : Trigonometry
  cos : Outport
  sin : Outport  Port=2
  wires:
  Gain/1 -> Cos1/1, Sin1/1
  Product1/1 -> Gain/1
  Sin1/1 -> sin/1
  clock/1 -> Product1/2
  freq/1 -> Product1/1
  Cos1/1 -> cos/1

== system HARMALYZE_model_simulink/Subsystem2/Subsystem9/An Bn finder ==
  signal : Inport
  pulse : Inport  Port=2
  cos : Inport  Port=3
  sin : Inport  Port=4
  "freq " : Inport  Port=5
  Add2 : Sum  Inputs=+-
  Constant1 : Constant  Value=0.0055
  Data Store Read1 : DataStoreRead  DataStoreName=simultion_time
  Product : Product  Inputs=3
  Product{1,3..5} (4 alike) : Product
  Product2 : Product  Inputs=3
  Pulse Generator1 : DiscretePulseGenerator  PulseType=Time based  Period=1  PulseWidth=0.01
  Transfer Fcn1 : TransferFcn  Numerator=[2]  Denominator=[1 0]
  Transfer Fcn2 : TransferFcn  Numerator=[2]  Denominator=[1 0]
  Variable Time Delay1 : VariableTransportDelay  MaximumDelay=10
  An : Outport
  Bn : Outport  Port=2
  wires:
  Product4/1 -> Bn/1
  Product5/1 -> An/1
  Product3/1 -> Product4/2  "Bn"
  Add2/1 -> Variable Time Delay1/2
  Variable Time Delay1/1 -> Product4/1, Product5/2
  Data Store Read1/1 -> Add2/1
  Constant1/1 -> Add2/2
  Product1/1 -> Product5/1  "An"
  Pulse Generator1/1 -> Variable Time Delay1/1
  "freq "/1 -> Product3/1, Product1/2
  Transfer Fcn1/1 -> Product1/1
  Transfer Fcn2/1 -> Product3/2
  sin/1 -> Product2/3
  cos/1 -> Product/3
  Product2/1 -> Transfer Fcn2/1
  Product/1 -> Transfer Fcn1/1
  signal/1 -> Product/2, Product2/1
  pulse/1 -> Product2/2, Product/1

== system HARMALYZE_model_simulink/Subsystem2/Subsystem9/magnitude ==
  An : Inport
  Bn : Inport  Port=2
  Add3 : Sum
  Math Function : Math  Operator=square  SignedPower=off  SaturateOnIntegerOverflow=on
  Math Function1 : Math  Operator=square  SignedPower=off  SaturateOnIntegerOverflow=on
  Sqrt : Sqrt  SaturateOnIntegerOverflow=on
  Out1 : Outport
  wires:
  An/1 -> Math Function/1
  Bn/1 -> Math Function1/1
  Sqrt/1 -> Out1/1
  Math Function1/1 -> Add3/2
  Add3/1 -> Sqrt/1
  Math Function/1 -> Add3/1

== system HARMALYZE_model_simulink/Subsystem2/Subsystem9/phase ==
  An : Inport
  Bn : Inport  Port=2
  Multiply1 : Gain  Gain=180/pi
  Sin : Trigonometry  Operator=atan2
  Out1 : Outport
  wires:
  Multiply1/1 -> Out1/1
  Bn/1 -> Sin/1
  An/1 -> Sin/2
  Sin/1 -> Multiply1/1

== system HARMALYZE_model_simulink/Subsystem2/Subsystem9/sin cos wave generator ==
  freq : Inport
  clock : Inport  Port=2
  Cos1 : Trigonometry  Operator=cos
  Gain : Gain  Gain=2*pi
  Product1 : Product
  Sin1 : Trigonometry
  cos : Outport
  sin : Outport  Port=2
  wires:
  Gain/1 -> Cos1/1, Sin1/1
  Product1/1 -> Gain/1
  Sin1/1 -> sin/1
  clock/1 -> Product1/2
  freq/1 -> Product1/1
  Cos1/1 -> cos/1
